simulink model "Kinematick"  (R2015b)
settings: Solver=VariableStepAuto  StartTime=0.0  StopTime=10.0  RelTol=1e-3
undefined symbols (not defined in the file): sigbuilder_block
libraries: simulink x3
settings Model: Creator=Druzhinin_Vasily  LastModifiedBy=User

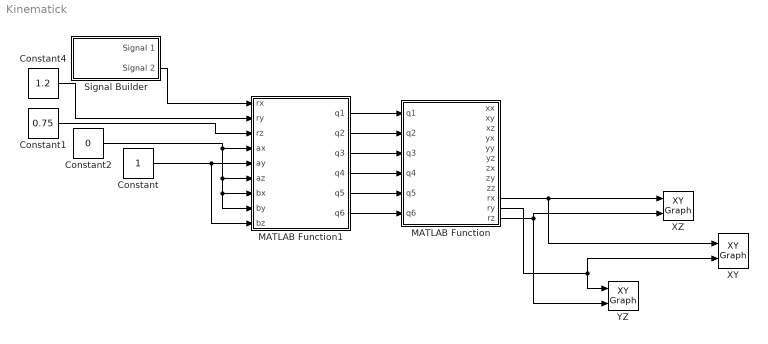
== system Kinematick ==
  Constant : Constant
  Constant1 : Constant  Value=0.75
  Constant2 : Constant  Value=0
  Constant4 : Constant  Value=1.2
  MATLAB Function : MATLAB Function  TreatAsAtomicUnit=on
  MATLAB Function1 : MATLAB Function  TreatAsAtomicUnit=on
  Signal Builder : Subsystem  Tag=STV Subsys  LoadFcn=sigbuilder_block('load',[183 267 550.5 336 ]);  StartFcn=sigbuilder_block('start');  StopFcn=sigbuilder_block('stop');  ClipboardFcn=sigbuilder_block('clipboard');  mask(Sigbuilder block){}
      mask help: Simulink:masks:SigbuilderBlock_MD
      mask init:
      | if ~strcmp(get_param(bdroot(gcbh),'SimulationStatus'),'stopped') tuvar = sigbuilder_block('maskInit'); end
      settings: CopyFcn=sigbuilder_block('copy');  DeleteFcn=sigbuilder_block('delete');  ModelCloseFcn=sigbuilder_block('modelClose');  PreSaveFcn=sigbuilder_block('preSave');  PauseFcn=sigbuilder_block('pause');  ContinueFcn=sigbuilder_block('continue');  NameChangeFcn=sigbuilder_block('namechange');  OpenFcn=sigbuilder_block('open',[183 267 550.5 336 ]);  CloseFcn=sigbuilder_block('close');
      mask Display: plot(0, 0, 100, 100,[2, 2, 32, 32, 2], [68, 8, 8, 68, 68],[32, 2], [38, 38], [32, 19, 2],[53, 60, 44], [32, 17, 17, 2],[16, 16, 31, 31]);txt = getActiveGroup(gcbh);text(2, 100, txt,'verticalAlignment', 'top');
  "XY " : simulink/Sinks/XY Graph  xmin=-0.5  xmax=1.5  ymin=-0.5  ymax=1.5  st=-1
  XZ : simulink/Sinks/XY Graph  xmin=-0.5  xmax=1.5  ymin=-0.5  ymax=1.5  st=-1
  "YZ " : simulink/Sinks/XY Graph  xmin=-0.5  xmax=1.5  ymin=-0.5  ymax=1.5  st=-1
  wires:
  Constant1/1 -> MATLAB Function1/3(rz)
  Constant2/1 -> MATLAB Function1/8(by), MATLAB Function1/7(bx), MATLAB Function1/6(az), MATLAB Function1/4(ax)
  Constant/1 -> MATLAB Function1/9(bz), MATLAB Function1/5(ay)
  Signal Builder/2(Signal 2) -> MATLAB Function1/1(rx)
  MATLAB Function1/2(q2) -> MATLAB Function/2(q2)
  MATLAB Function1/1(q1) -> MATLAB Function/1(q1)
  MATLAB Function1/3(q3) -> MATLAB Function/3(q3)
  MATLAB Function1/4(q4) -> MATLAB Function/4(q4)
  MATLAB Function1/5(q5) -> MATLAB Function/5(q5)
  MATLAB Function1/6(q6) -> MATLAB Function/6(q6)
  MATLAB Function/12(rz) -> "YZ "/2, XZ/2
  MATLAB Function/10(rx) -> "XY "/1, XZ/1
  MATLAB Function/11(ry) -> "YZ "/1, "XY "/2
  Constant4/1 -> MATLAB Function1/2(ry)

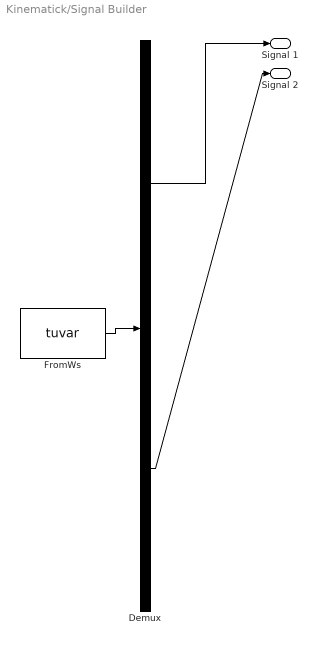
== system Kinematick/Signal Builder ==
  Demux : Demux  Tag=STV Demux  Outputs=2
  FromWs : FromWorkspace  Tag=STV FromWs  VariableName=tuvar  SampleTime=0
      SigBuilderData=|
      | common.afterFinalStr = 'Extrapolate'
      | common.sampleTime = 0
      | dataSet.timeRange = [0 10]
      | dataSet.name = 'Group 1'
      | sbobj.Groups.Name = 'Group 1'
      | sbobj.Groups.Signals(1).Name = 'Signal 1'
      | sbobj.Groups.Signals(1).XData = [0 4 4 6 6 10]
      | sbobj.Groups.Signals(1).YData = [0.4 0.4 1 1 1.4 1.4]
      | sbobj.Groups.Signals(2).Name = 'Signal 2'
      | sbobj.Groups.Signals(2).XData = [0 5 5 10]
      | sbobj.Groups.Signals(2).YData = [-0.3 0 0.2 0.7]
  Signal 1 : Outport  Tag=STV Outport
  Signal 2 : Outport  Tag=STV Outport  Port=2
  wires:
  Demux/1 -> Signal 1/1
  FromWs/1 -> Demux/1
  Demux/2 -> Signal 2/1

== matlab function Kinematick/MATLAB Function1 ==
  data: q1 output; q2 output; q3 output; q4 output; q5 output; q6 output; rx input; ry input; rz input; ax input; ay input; az input; bx input; by input; bz input
function [q1,q2,q3,q4,q5,q6] = fcn(rx,ry,rz,ax,ay,az,bx,by,bz)

    % РћР—Рљ РґР»СЏ 6С‚Рё СЃС‚РµРїРµРЅРЅРѕРіРѕ РњРњ. 
    pi = 3.14159265358979;
    % Р”Р»РёРЅС‹ Р·РІРµРЅСЊРµРІ.
    L1 = 0.4;
    L2 = 0.7;
    L3 = 0.7;
    L4 = 0.1;
    
    % РћРіСЂР°РЅРёС‡РµРЅРёСЏ РїРѕ СЃС‚РµРїРµРЅСЏРј РїРѕРґРІРёР¶РЅРѕСЃС‚Рё. 
    % -pi/2 < qi < pi/2
    % -pi/2 < fi < pi/2, РіРґРµ fi=q2+q3
    
    Rx = rx-ax*L4;
    Ry = ry-ay*L4;
    Rz = rz-az*L4;
 
  if (Ry==0) Ry = 0.0000001; end;  
  q1 = -atan(Rx/Ry);
  
    f1 = (Rz-L1)/L3;
    f2 = -L2/L3;
    f3 = Ry/(L3*cos(q1));
    
    g1 = 2*f1*f2;
    g2 = 2*f2*f3;
    g3 = 1-f1*f1-f2*f2-f3*f3;
           
  q2 = asin(g3/sqrt(g1*g1+g2*g2)) - atan(f3/f1); 
    if (q2<-pi/2) q2 = q2+pi; end; % 
  q3 = asin(f1+f2*sin(q2)) - q2;   
  
    fi  = q2+q3;  
    sfi = sin(fi);
    cfi = cos(fi);
    if (ay==0) ay = 0.0000001; end;  
    alfa = -q1 - atan(ax/ay); 
    if (abs(alfa)<0.0000001) alfa = 0; end;

  if (alfa >= 0) q5 =  acos(-ax*sin(q1)*cfi + ay*cos(q1)*cfi + az*sfi); 
  else           q5 = -acos(-ax*sin(q1)*cfi + ay*cos(q1)*cfi + az*sfi);
  end;                                                                 
  
    k = az - sfi*cos(q5);

  if (q5==0) q5 = 0.0000001; end;
  q4 = acos((-ax*cos(q1)-ay*sin(q1))/sin(q5));
  if (k  < 0) q4 = -q4; end; 
  if (q5 < 0) q4 = -q4; end; 
    
    gammax =  bz*(sin(q1)*sin(q4) - cos(q1)*sfi*cos(q4)) - by*cfi*cos(q4);
    gammay = -bz*(cos(q1)*sin(q4) + sin(q1)*sfi*cos(q4)) + bx*cfi*cos(q4);
    
    betta = gammax*ax + gammay*ay;
    
  q6 = acos(  bx*(cos(q1)*sin(q4)+sin(q1)*sfi*cos(q4))  +  by*(sin(q1)*sin(q4)-cos(q1)*sfi*cos(q4))  +  bz*(cfi*cos(q4))  );
  if (betta<0)  q6 = -q6; end; 
  
  if (q1<-pi/2) q1 = -pi/2; end; 
  if (q1> pi/2) q1 =  pi/2; end;
  if (q2<-pi/2) q2 = -pi/2; end; 
  if (q2> pi/2) q2 =  pi/2; end;
  if (q3<-pi/2) q3 = -pi/2; end; 
  if (q3> pi/2) q3 =  pi/2; end;
  if (q4<-pi/2) q4 = -pi/2; end; 
  if (q4> pi/2) q4 =  pi/2; end;
  if (q5<-pi/2) q5 = -pi/2; end; 
  if (q5> pi/2) q5 =  pi/2; end;
  if (q6<-pi/2) q6 = -pi/2; end; 
  if (q6> pi/2) q6 =  pi/2; end;
  
end

== matlab function Kinematick/MATLAB Function ==
  data: q1 input; xx output; q2 input; q3 input; q4 input; q5 input; q6 input; xy output; xz output; yx output; yy output; yz output; zx output; zy output; zz output; rx output; ry output; rz output
function [xx,xy,xz,yx,yy,yz,zx,zy,zz,rx,ry,rz] = fcn(q1,q2,q3,q4,q5,q6)

    L1 = 0.4;
    L2 = 0.7;
    L3 = 0.7;
    L4 = 0.1;
    
  % =======================================================================
  
  s1  = sin(q1);
  s2  = sin(q2);
  s3  = sin(q3);
  s4  = sin(q4);
  s5  = sin(q5);
  s6  = sin(q6);  
  c1  = cos(q1);
  c2  = cos(q2);
  c3  = cos(q3);
  c4  = cos(q4);
  c5  = cos(q5);
  c6  = cos(q6);
  sfi = sin(q2+q3);
  cfi = cos(q2+q3);
  
  A1 = [ (-s1) 0     c1    0     ; c1    0  s1 0     ; 0 1 0 L1 ; 0 0 0 1 ];
  A2 = [ c2    (-s2) 0     L2*c2 ; s2    c2 0  L2*s2 ; 0 0 1 0  ; 0 0 0 1 ];
  A3 = [ (-s3) 0     c3    0     ; c3    0  s3 0     ; 0 1 0 0  ; 0 0 0 1 ];
  A4 = [ (-s4) 0     c4    0     ; c4    0  s4 0     ; 0 1 0 L3 ; 0 0 0 1 ];
  A5 = [ (-c5) 0     (-s5) 0     ; (-s5) 0  c5 0     ; 0 1 0 0  ; 0 0 0 1 ];
  A6 = [ c6   (-s6)  0     0     ; s6    c6 0  0     ; 0 0 1 L4 ; 0 0 0 1 ];
  
  T = A1*A2*A3*A4*A5*A6;
  
  xx = T(1,1);
  xy = T(2,1);
  xz = T(3,1);
  yx = T(1,2);
  yy = T(2,2);
  yz = T(3,2);
  zx = T(1,3);
  zy = T(2,3);
  zz = T(3,3);
  rx = T(1,4);
  ry = T(2,4);
  rz = T(3,4);
  
  % СЃС‚СЂ. 202 ("РЎРёСЃС‚РµРјС‹ СѓРїСЂР°РІР»РµРЅРёСЏ РїРѕРґРІРѕРґРЅС‹РјРё СЂРѕР±РѕС‚Р°РјРё" - Р·РµР»РµРЅР°СЏ РєРЅРёРіР°)
  % | xx yx zx rx |         
  % | xy yy zy ry |         [ xy yy zy ] = B
  % | xz yz zz rz |         [ xz yz zz ] = A
  % | 0  0  0  1  |, РіРґРµ    [ rx ry rz ] = [ x  y  z ]
  
end
